simulink library "pathFollowingCtrlAoATurbFault_cl"  (R2020a)
settings: Solver=VariableStepAuto  StartTime=0.0  StopTime=10.0  RelTol=1e-3
undefined symbols (not defined in the file or in its folder): env, FLIGHTCONTROLLER, fltCtrl, initializeBussesFromBlock, lapN, pthCtrl1, rollVec, timeVec, tSwitch, VEHICLE, vhcl, yawVec
libraries: simulink x9, filteredPIDController_ul x4, vrlib x3, eulAng2RotMat_ul x2, alphaBeta_ul x2, velocityAngle_ul x2, filteredPIDControllerAWGS_ul x1, stopwatch_ul x1, tensionLimitCtrl_cl x1, courseFollowExp_cl x1, ctrlAllocMatrix3Comp_cl x1, angleBtw2Vecs_ul x1
settings Model: Creator=jldanie5  LastModifiedBy=andre
settings DataIOCC: ReturnWorkspaceOutputs=off
settings DebuggingCC: ArithmeticOperatorsInVariantConditions=warning
settings SFSimCC: CustomCodeUndefinedFunction=UseInterfaceOnly

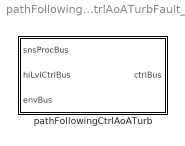
== system pathFollowingCtrlAoATurbFault_cl ==
  pathFollowingCtrlAoATurb : Subsystem  LoadFcn=initializeBussesFromBlock(gcb)  InitFcn=initializeBussesFromBlock(gcb)  StartFcn=initializeBussesFromBlock(gcb)  VariantControl=strcmpi(FLIGHTCONTROLLER,'pathFollowingControllerManta')  mask{initPosForInitSStar=vhcl.initPosVecGnd.Value, fluidDensity=env.water.density.Value, pathCtrl=pthCtrl1, aeroStruct=vhcl.struct('OCT.aeroSurf')}
      mask prompts: initPosForInitSStar "Initial Position"; fluidDensity "Fluid Density"; pathCtrl "Controller"; aeroStruct "Aerodynamic Structure"
      settings: MinAlgLoopOccurrences=on
      mask DialogControl Container3 Prompt: courseFollow Params
      mask DialogControl Container4 Prompt: setpointToOutput Params

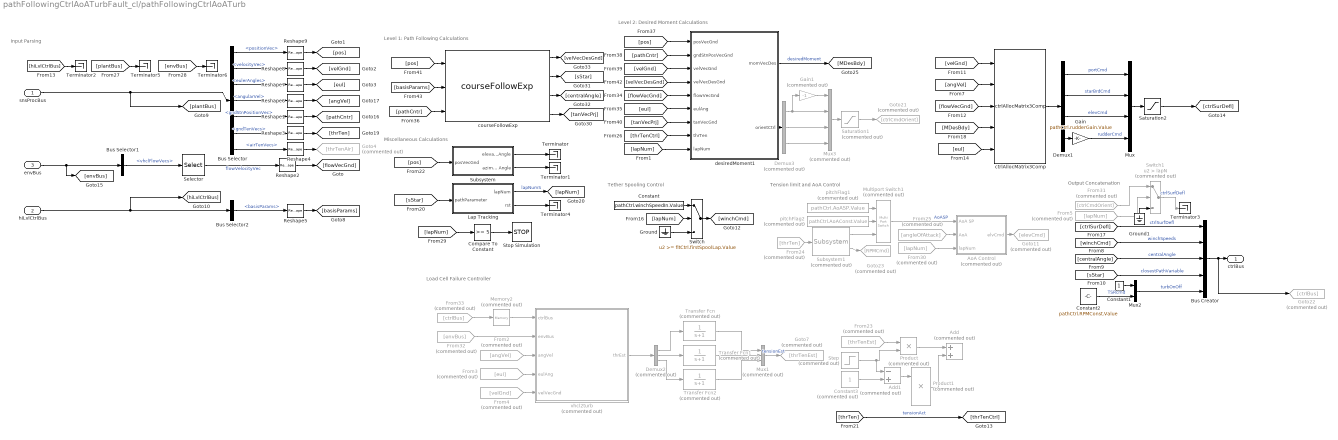
== system pathFollowingCtrlAoATurbFault_cl/pathFollowingCtrlAoATurb ==
  note: Load Cell Failure Controller
  note: Tension limit and AoA Control
  note: Miscellaneous Calculations
  note: Output Concatenation
  note: Tether Spooling Control
  note: Input Parsing
  note: Level 1: Path Following Calculations
  note: Level 2: Desired Moment Calculations
  snsProcBus : Inport  OutDataTypeStr=Bus: sensorsProcessingBus
  hiLvlCtrlBus : Inport  Port=2  OutDataTypeStr=Bus: hiLvlCtrlBus
  envBus : Inport  Port=3  OutDataTypeStr=Bus: envBus
  Add : Sum  Commented=on
  Add1 : Sum  Commented=on  Inputs=-+
  AoA Control : Subsystem  Commented=on
  Bus Creator : BusCreator  Inputs=5
  Bus Selector : BusSelector  OutputSignals=positionVec,velocityVec,eulerAngles,angularVel,gndStnPositionVec,gndTenVecs,airTenVecs
  Bus Selector1 : BusSelector  OutputSignals=vhclFlowVecs
  Bus Selector2 : BusSelector  OutputSignals=basisParams
  Compare To Constant : simulink/Logic and Bit Operations/Compare To Constant  relop=>=  const=5  OutDataTypeStr=boolean
  Constant : Constant  Value=pathCtrl.winchSpeedIn.Value
  Constant1 : Constant
  Constant2 : Constant  Value=pathCtrl.RPMConst.Value
  Constant3 : Constant  Commented=on
  Demux1 : Demux
  Demux2 : Demux  Commented=on  Outputs=3
  Demux3 : Demux  Commented=on  Outputs=3
  From2 : From  Commented=on  GotoTag=angVel
  From23 : From  Commented=on  GotoTag=thrTenEst
  From24 : From  Commented=on  GotoTag=thrTen
  From25 : From  Commented=on  GotoTag=angleOfAttack
  From3 : From  Commented=on  GotoTag=eul
  From30 : From  Commented=on  GotoTag=lapNum
  From31 : From  Commented=on  GotoTag=ctrlCmdOrient
  From32 : From  Commented=on  GotoTag=envBus
  From33 : From  Commented=on  GotoTag=ctrlBus
  From4 : From  Commented=on  GotoTag=velGnd
  From5 : From  Commented=on  GotoTag=lapNum
  Gain : Gain  Gain=pathCtrl.rudderGain.Value
  Gain1 : Gain  Commented=on  Gain=-1
  Goto11 : Goto  Commented=on  GotoTag=elevCmd
  Goto21 : Goto  Commented=on  GotoTag=ctrlCmdOrient
  Goto22 : Goto  Commented=on  GotoTag=ctrlBus
  Goto23 : Goto  Commented=on  GotoTag=RPMCmd
  Goto4 : Goto  Commented=on  GotoTag=thrTenAir
  Goto7 : Goto  Commented=on  GotoTag=thrTenEst
  Ground : Ground
  Ground1 : Ground
  Lap Tracking : Subsystem
  Memory2 : Memory  Commented=on  InitialCondition=pathCtrl.initPathVar.Value
  Multiport Switch1 : MultiPortSwitch  Commented=on  DataPortOrder=Specify indices  Inputs=2  DataPortIndices={0,1}
  Mux : Mux
  Mux1 : Mux  Commented=on  Inputs=3
  Mux2 : Mux  Inputs=2
  Mux3 : Mux  Commented=on
  Product : Product  Commented=on
  Product1 : Product  Commented=on
  Reshape{1..9} (9 alike) : Reshape  OutputDimensionality=Column vector (2-D)
  Saturation1 : Saturate  Commented=on  UpperLimit=pathCtrl.controlSigMax.upperLimit.Value  LowerLimit=pathCtrl.controlSigMax.lowerLimit.Value
  Saturation2 : Saturate  UpperLimit=pathCtrl.controlSigMax.upperLimit.Value  LowerLimit=pathCtrl.controlSigMax.lowerLimit.Value
  Selector : Selector  NumberOfDimensions=2  InputPortWidth=3  IndexOptions=Select all,Index vector (dialog)  Indices=[1 3],5  OutputSizes=1,1
  Step : Step  Commented=on  Time=tSwitch  SampleTime=0
  Stop Simulation : Stop
  Subsystem : Subsystem
  Subsystem1 : tensionLimitCtrl_cl/Subsystem  Commented=on  SystemSampleTime=-1  Latency=0  AutoFrameSizeCalculation=off
  Switch : Switch  Threshold=fltCtrl.firstSpoolLap.Value
  Switch1 : Switch  Commented=on  Criteria=u2 > Threshold  Threshold=lapN
  Terminator{,1..6} (7 alike) : Terminator
  Transfer Fcn : TransferFcn  Commented=on  Denominator=[1 1]
  Transfer Fcn1 : TransferFcn  Commented=on  Denominator=[1 1]
  Transfer Fcn2 : TransferFcn  Commented=on  Denominator=[1 1]
  courseFollowExp : courseFollowExp_cl/courseFollowExp  SystemSampleTime=-1  Latency=0  AutoFrameSizeCalculation=off
  ctrlAllocMatrix3Comp : ctrlAllocMatrix3Comp_cl/ctrlAllocMatrix3Comp  aeroStruct=vhcl.struct('OCT.aeroSurf')  fluidDensity=fluidDensity  arms=vhcl.struct('OCT.thrAttch')
  desiredMoment1 : Subsystem
  pitchFlag1 : Constant  Commented=on  Value=pathCtrl.AoASP.Value
  pitchFlag2 : Constant  Commented=on  Value=pathCtrl.AoAConst.Value
  vhcl2turb : Subsystem  Commented=on  VariantControl=strcmpi(VEHICLE,'vhcl2turb')  mask{vcl=vhcl, rho=env.water.density.Value, grav=env.gravAccel.Value}
      mask prompts: vcl "Vehicle"; rho "Density"; grav "Gravity"
      mask DialogControl Container9 Prompt: General
      mask DialogControl Container5 Prompt: Vehicle object (OCT.vehicle)
      mask DialogControl ParameterGroupVar Prompt: Environment Object (OCT.env)
      mask Display:
      | image('kite2.PNG',[0 0 700 700]/4,'on')
      | 
      | port_label('input',1,'ctrlBus')
      | port_label('input',2,'envBus')
      | port_label('input',3,'nodeForceVecs')
      | 
      | port_label('output',1,'thrTension')
  ctrlBus : Outport  OutDataTypeStr=Bus: fltCtrlBus  VectorParamsAs1DForOutWhenUnconnected=off
  wires:
  Bus Selector/6 -> Reshape3/1  "<gndTenVecs>"
  Reshape3/1 -> [thrTen]
  snsProcBus/1 -> Bus Selector/1, [plantBus]
  Bus Selector/2 -> Reshape8/1  "<velocityVec>"
  Bus Selector/1 -> Reshape9/1  "<positionVec>"
  Bus Selector/3 -> Reshape7/1  "<eulerAngles>"
  Bus Creator/1 -> Goto22/1, ctrlBus/1
  [winchCmd] -> Bus Creator/2  "winchSpeeds"
  hiLvlCtrlBus/1 -> [hiLvlCtrlBus], Bus Selector2/1
  [centralAngle] -> Bus Creator/3  "centralAngle"
  [sStar] -> Bus Creator/4  "closestPathVariable"
  Bus Selector/4 -> Reshape6/1  "<angularVel>"
  [angVel] -> ctrlAllocMatrix3Comp/2
  [velGnd] -> ctrlAllocMatrix3Comp/1
  [flowVecGnd] -> ctrlAllocMatrix3Comp/3
  Demux1/1 -> Mux/1  "portCmd"
  Demux1/2 -> Mux/2  "starBrdCmd"
  [MDesBdy] -> ctrlAllocMatrix3Comp/4
  [ctrlSurDefl] -> Bus Creator/1  "ctrlSurfDefl"
  Bus Selector2/1 -> Reshape5/1  "<basisParams>"
  Reshape5/1 -> [basisParams]
  Saturation2/1 -> [ctrlSurDefl]
  Reshape2/1 -> [flowVecGnd]
  Reshape6/1 -> [angVel]
  Reshape7/1 -> [eul]
  Reshape8/1 -> [velGnd]
  Reshape9/1 -> [pos]
  [eul] -> ctrlAllocMatrix3Comp/5
  Selector/1 -> Reshape2/1  "flowVelocityVec"
  envBus/1 -> [envBus], Bus Selector1/1
  Bus Selector1/1 -> Selector/1  "<vhclFlowVecs>"
  Reshape1/1 -> [pathCntr]
  Bus Selector/5 -> Reshape1/1  "<gndStnPositionVec>"
  Demux1/4 -> Gain/1
  [pos] -> Subsystem/1(posVecGnd)
  Subsystem/1(elevationAngle) -> Terminator/1
  Subsystem/2(azimuth Angle) -> Terminator1/1
  [sStar] -> Lap Tracking/1(pathParameter)
  Lap Tracking/2(rst) -> Terminator4/1
  Lap Tracking/1(lapNum) -> [lapNum]  "lapNumS"
  [plantBus] -> Terminator5/1
  [envBus] -> Terminator6/1
  Switch/1 -> [winchCmd]
  [lapNum] -> Switch/2
  Constant/1 -> Switch/1
  Ground/1 -> Switch/3
  [lapNum] -> Compare To Constant/1
  Compare To Constant/1 -> Stop Simulation/1
  ctrlAllocMatrix3Comp/1 -> Demux1/1
  Gain/1 -> Mux/4  "rudderCmd"
  [hiLvlCtrlBus] -> Terminator2/1
  From30/1 -> AoA Control/3(lapNum)
  AoA Control/1(elvCmd) -> Goto11/1
  From25/1 -> AoA Control/2(AoA)
  Mux/1 -> Saturation2/1
  Subsystem1/1 -> Multiport Switch1/3
  pitchFlag2/1 -> Multiport Switch1/2
  pitchFlag1/1 -> Multiport Switch1/1
  From24/1 -> Subsystem1/1
  Multiport Switch1/1 -> AoA Control/1(AoA SP)  "AoASP"
  Subsystem1/2 -> Goto23/1
  Mux2/1 -> Bus Creator/5  "turbOnOff"
  Constant1/1 -> Mux2/1
  Constant2/1 -> Mux2/2  "TSRcmd"
  Demux1/3 -> Mux/3  "elevCmd"
  [velVecDesGnd] -> desiredMoment1/4(velVecDesGnd)
  [velGnd] -> desiredMoment1/3(velVecGnd)
  [eul] -> desiredMoment1/6(eulAng)
  [basisParams] -> courseFollowExp/2
  [pathCntr] -> desiredMoment1/2(gndStnPosVecGnd)
  courseFollowExp/2 -> [sStar]
  [pos] -> desiredMoment1/1(posVecGnd)
  [tanVecPrj] -> desiredMoment1/7(tanVecGnd)
  [pathCntr] -> courseFollowExp/3
  desiredMoment1/1(momVecDes) -> [MDesBdy]  "desiredMoment"
  [pos] -> courseFollowExp/1
  courseFollowExp/3 -> [centralAngle]
  courseFollowExp/4 -> [tanVecPrj]
  courseFollowExp/1 -> [velVecDesGnd]
  [flowVecGnd] -> desiredMoment1/5(flowVecGnd)
  [thrTenCtrl] -> desiredMoment1/8(thrTen)
  Reshape4/1 -> Goto4/1
  Bus Selector/7 -> Reshape4/1  "<airTenVecs>"
  From23/1 -> Product/1
  [thrTen] -> [thrTenCtrl]  "tensionAct"
  Step/1 -> Product/2, Add1/1
  Product/1 -> Add/1
  Constant3/1 -> Add1/2
  Add1/1 -> Product1/1
  Product1/1 -> Add/2
  Mux1/1 -> Goto7/1  "tensionEst"
  Demux2/1 -> Transfer Fcn/1
  Demux2/2 -> Transfer Fcn1/1
  Demux2/3 -> Transfer Fcn2/1
  Transfer Fcn/1 -> Mux1/1
  Transfer Fcn1/1 -> Mux1/2
  Transfer Fcn2/1 -> Mux1/3
  desiredMoment1/2(orientCtrl) -> Demux3/1
  Demux3/1 -> Gain1/1, Mux3/2
  Gain1/1 -> Mux3/1
  Demux3/2 -> Mux3/3
  Mux3/1 -> Saturation1/1
  From31/1 -> Switch1/1
  From5/1 -> Switch1/2
  Switch1/1 -> Terminator3/1  "ctrlSurfDefl"
  Saturation1/1 -> Goto21/1
  From32/1 -> vhcl2turb/2(envBus)
  From33/1 -> Memory2/1
  Memory2/1 -> vhcl2turb/1(ctrlBus)
  vhcl2turb/1(thrEst) -> Demux2/1
  From2/1 -> vhcl2turb/3(angVel)
  From3/1 -> vhcl2turb/4(eulAng)
  From4/1 -> vhcl2turb/5(velVecGnd)
  Demux3/3 -> Mux3/4
  [lapNum] -> desiredMoment1/9(lapNum)
  Ground1/1 -> Switch1/3

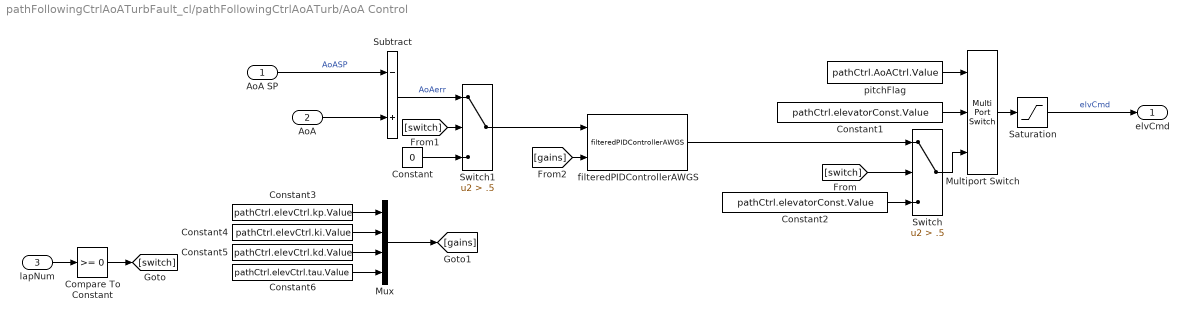
== system pathFollowingCtrlAoATurbFault_cl/pathFollowingCtrlAoATurb/AoA Control ==
  AoA SP : Inport
  AoA : Inport  Port=2
  lapNum : Inport  Port=3
  Compare To Constant : simulink/Logic and Bit Operations/Compare To Constant  relop=>=  const=0  OutDataTypeStr=boolean
  Constant : Constant  Value=0
  Constant1 : Constant  Value=pathCtrl.elevatorConst.Value
  Constant2 : Constant  Value=pathCtrl.elevatorConst.Value
  Constant3 : Constant  Value=pathCtrl.elevCtrl.kp.Value
  Constant4 : Constant  Value=pathCtrl.elevCtrl.ki.Value
  Constant5 : Constant  Value=pathCtrl.elevCtrl.kd.Value
  Constant6 : Constant  Value=pathCtrl.elevCtrl.tau.Value
  Multiport Switch : MultiPortSwitch  DataPortOrder=Specify indices  Inputs=2  DataPortIndices={0,1}
  Mux : Mux
  Saturation : Saturate  UpperLimit=pathCtrl.elevCtrlMax.upperLimit.Value  LowerLimit=pathCtrl.elevCtrlMax.lowerLimit.Value
  Subtract : Sum  Inputs=-+
  Switch : Switch  Criteria=u2 > Threshold  Threshold=.5
  Switch1 : Switch  Criteria=u2 > Threshold  Threshold=.5
  filteredPIDControllerAWGS : filteredPIDControllerAWGS_ul/filteredPIDControllerAWGS  cmax=pathCtrl.elevCtrlMax.upperLimit.Value  cmin=pathCtrl.elevCtrlMax.lowerLimit.Value
  pitchFlag : Constant  Value=pathCtrl.AoACtrl.Value
  elvCmd : Outport
  wires:
  AoA/1 -> Subtract/2
  Constant1/1 -> Multiport Switch/2
  pitchFlag/1 -> Multiport Switch/1
  AoA SP/1 -> Subtract/1  "AoASP"
  Multiport Switch/1 -> Saturation/1
  Constant2/1 -> Switch/3
  Saturation/1 -> elvCmd/1  "elvCmd"
  lapNum/1 -> Compare To Constant/1
  Compare To Constant/1 -> [switch]
  [switch] -> Switch/2
  Subtract/1 -> Switch1/1  "AoAerr"
  [switch] -> Switch1/2
  Constant/1 -> Switch1/3
  Switch/1 -> Multiport Switch/3
  Switch1/1 -> filteredPIDControllerAWGS/1
  filteredPIDControllerAWGS/1 -> Switch/1
  [gains] -> filteredPIDControllerAWGS/2
  Mux/1 -> [gains]
  Constant3/1 -> Mux/1
  Constant4/1 -> Mux/2
  Constant5/1 -> Mux/3
  Constant6/1 -> Mux/4

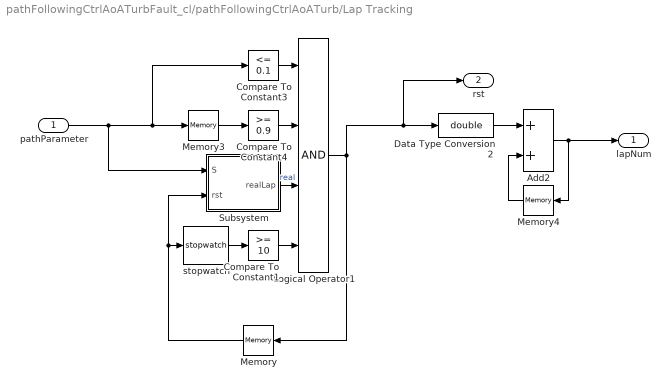
== system pathFollowingCtrlAoATurbFault_cl/pathFollowingCtrlAoATurb/Lap Tracking ==
  pathParameter : Inport
  Add2 : Sum
  Compare To Constant1 : simulink/Logic and Bit Operations/Compare To Constant  relop=>=  const=10  OutDataTypeStr=boolean
  Compare To Constant3 : simulink/Logic and Bit Operations/Compare To Constant  relop=<=  const=0.1  OutDataTypeStr=boolean
  Compare To Constant4 : simulink/Logic and Bit Operations/Compare To Constant  relop=>=  const=0.9  OutDataTypeStr=boolean
  Data Type Conversion2 : DataTypeConversion  OutDataTypeStr=double
  Logical Operator1 : Logic  Inputs=4  AllPortsSameDT=off  OutDataTypeStr=boolean
  Memory : Memory  InitialCondition=false
  Memory3 : Memory
  Memory4 : Memory
  Subsystem : Subsystem
  stopwatch : stopwatch_ul/stopwatch  SystemSampleTime=-1  Latency=0  AutoFrameSizeCalculation=off
  lapNum : Outport  VectorParamsAs1DForOutWhenUnconnected=off
  rst : Outport  Port=2  VectorParamsAs1DForOutWhenUnconnected=off
  wires:
  Compare To Constant3/1 -> Logical Operator1/1
  Memory3/1 -> Compare To Constant4/1
  Data Type Conversion2/1 -> Add2/1
  Logical Operator1/1 -> rst/1, Data Type Conversion2/1, Memory/1
  Memory4/1 -> Add2/2
  Add2/1 -> lapNum/1, Memory4/1
  Compare To Constant4/1 -> Logical Operator1/2
  pathParameter/1 -> Subsystem/1(S), Compare To Constant3/1, Memory3/1
  stopwatch/1 -> Compare To Constant1/1
  Memory/1 -> Subsystem/2(rst), stopwatch/1
  Compare To Constant1/1 -> Logical Operator1/4
  Subsystem/1(realLap) -> Logical Operator1/3  "real"

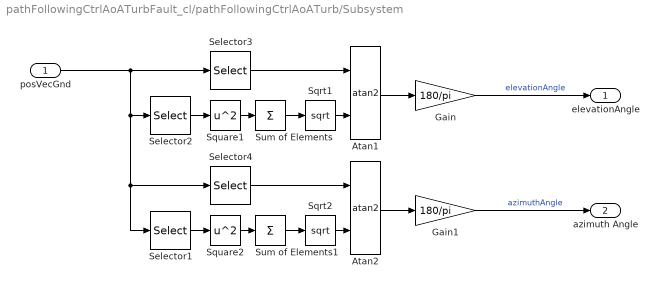
== system pathFollowingCtrlAoATurbFault_cl/pathFollowingCtrlAoATurb/Subsystem ==
  posVecGnd : Inport
  Atan1 : Trigonometry  Operator=atan2
  Atan2 : Trigonometry  Operator=atan2
  Gain : Gain  Gain=180/pi
  Gain1 : Gain  Gain=180/pi
  Selector1 : Selector  InputPortWidth=3  IndexOptions=Index vector (dialog)  Indices=1  OutputSizes=1
  Selector2 : Selector  InputPortWidth=3  IndexOptions=Index vector (dialog)  Indices=[1 2]  OutputSizes=1
  Selector3 : Selector  InputPortWidth=3  IndexOptions=Index vector (dialog)  Indices=3  OutputSizes=1
  Selector4 : Selector  InputPortWidth=3  IndexOptions=Index vector (dialog)  Indices=2  OutputSizes=1
  Sqrt1 : Sqrt  SaturateOnIntegerOverflow=on
  Sqrt2 : Sqrt  SaturateOnIntegerOverflow=on
  Square1 : Math  Operator=square  SignedPower=on  SaturateOnIntegerOverflow=on
  Square2 : Math  Operator=square  SignedPower=on  SaturateOnIntegerOverflow=on
  Sum of Elements : Sum  Inputs=+
  Sum of Elements1 : Sum  Inputs=+
  elevationAngle : Outport
  azimuth Angle : Outport  Port=2
  wires:
  Sqrt1/1 -> Atan1/2
  Square1/1 -> Sum of Elements/1
  Selector3/1 -> Atan1/1
  Sum of Elements/1 -> Sqrt1/1
  Atan1/1 -> Gain/1
  Selector2/1 -> Square1/1
  Gain/1 -> elevationAngle/1  "elevationAngle"
  Atan2/1 -> Gain1/1
  Square2/1 -> Sum of Elements1/1
  Sum of Elements1/1 -> Sqrt2/1
  Selector1/1 -> Square2/1
  posVecGnd/1 -> Selector1/1, Selector4/1, Selector2/1, Selector3/1
  Sqrt2/1 -> Atan2/2
  Selector4/1 -> Atan2/1
  Gain1/1 -> azimuth Angle/1  "azimuthAngle"

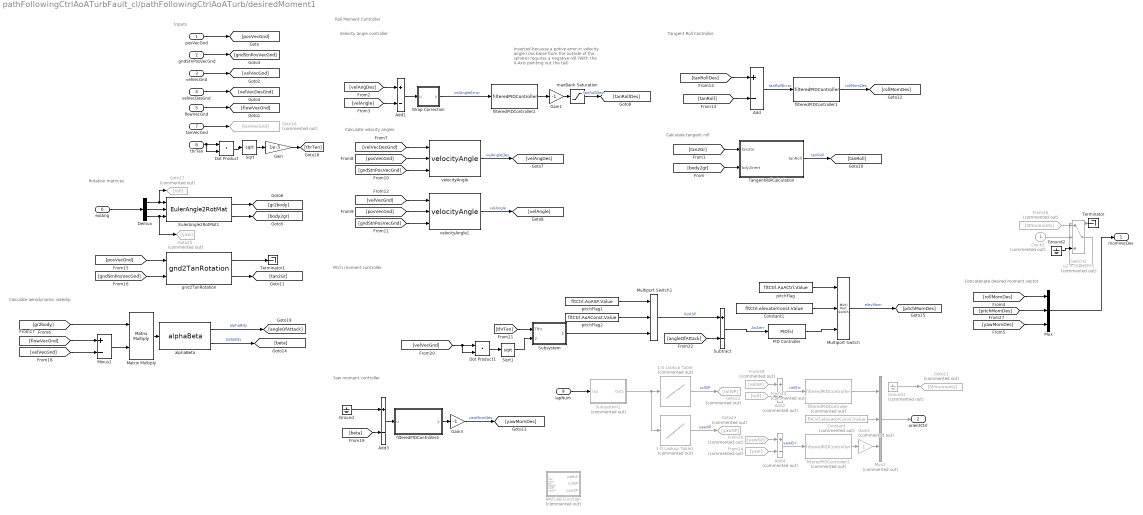
== system pathFollowingCtrlAoATurbFault_cl/pathFollowingCtrlAoATurb/desiredMoment1 ==
  note: Roll Moment Controller
  note: Calculate aerodynamic sideslip
  note: Concatenate desired moment vector
  note: Tangent Roll Controller
  note: Calculate tangent roll
  note: Calculate velocity angles
  note: Rotation matrices
  note: Inputs
  note: Velocity angle controller
  note: Inverted because a potive error
      | in velocity angle (clockwise from the
      | outside of the sphere) requires a negative
      | roll (With the X-Axis pointing out the tail)
  note: Pitch moment controller
  note: Yaw moment controller
  posVecGnd : Inport
  gndStnPosVecGnd : Inport  Port=2
  velVecGnd : Inport  Port=3
  velVecDesGnd : Inport  Port=4
  flowVecGnd : Inport  Port=5
  eulAng : Inport  Port=6
  tanVecGnd : Inport  Port=7
  thrTen : Inport  Port=8
  lapNum : Inport  Port=9
  1-D Lookup Table : Lookup_n-D  Commented=on  NumberOfTableDimensions=1  BreakpointsForDimension1=timeVec  Table=rollVec  InternalRulePriority=Speed  RndMeth=Simplest  InputSameDT=on
  1-D Lookup Table1 : Lookup_n-D  Commented=on  NumberOfTableDimensions=1  BreakpointsForDimension1=timeVec  Table=yawVec  InternalRulePriority=Speed  RndMeth=Simplest  InputSameDT=on
  Add : Sum  Inputs=+-
  Add1 : Sum  Inputs=+-
  Add2 : Sum  Commented=on  Inputs=+-
  Add3 : Sum  Inputs=+-
  Add4 : Sum  Commented=on  Inputs=+-
  Clock2 : Clock  Commented=on
  Constant : Constant  Commented=on  Value=fltCtrl.elevatorConst.Value
  Constant1 : Constant  Value=fltCtrl.elevatorConst.Value
  Demux : Demux  Outputs=3
  Dot Product : DotProduct  InputSameDT=on  OutDataTypeStr=Inherit: Inherit via internal rule
  Dot Product1 : DotProduct  InputSameDT=on  OutDataTypeStr=Inherit: Inherit via internal rule
  EulerAngle2RotMat1 : eulAng2RotMat_ul/EulerAngle2RotMat  SystemSampleTime=-1  Latency=0  AutoFrameSizeCalculation=off
  From23 : From  Commented=on  GotoTag=roll
  From24 : From  Commented=on  GotoTag=yaw
  From26 : From  Commented=on  GotoTag=SPmoments
  From28 : From  Commented=on  GotoTag=rollSP
  From29 : From  Commented=on  GotoTag=yawSP
  Gain : Gain  Gain=1e-3
  Gain1 : Gain  Gain=-1
  Gain3 : Gain  Gain=-1
  Gain5 : Gain  Commented=on  Gain=-1
  Goto16 : Goto  Commented=on  GotoTag=tanVecGnd
  Goto17 : Goto  Commented=on  GotoTag=roll
  Goto20 : Goto  Commented=on  GotoTag=yaw
  Goto21 : Goto  Commented=on  GotoTag=SPmoments
  Goto22 : Goto  Commented=on  GotoTag=rollSP
  Goto23 : Goto  Commented=on  GotoTag=yawSP
  Ground : Ground
  Ground1 : Ground  Commented=on
  Ground2 : Ground
  MATLAB Function : MATLAB Function  Commented=on  TreatAsAtomicUnit=on
  Matrix Multiply : Product  Multiplication=Matrix(*)
  Minus1 : Sum  Inputs=+-
  Multiport Switch : MultiPortSwitch  DataPortOrder=Specify indices  Inputs=2  DataPortIndices={0,1}
  Multiport Switch1 : MultiPortSwitch  DataPortOrder=Specify indices  Inputs=2  DataPortIndices={0,1}
  Mux : Mux  Inputs=3
  Mux2 : Mux  Commented=on  Inputs=3
  PID Controller : simulink/Continuous/PID Controller  Controller=PID  Form=Parallel  TimeDomain=Continuous-time  UseExternalTs=off  SampleTime=-1  IntegratorMethod=Forward Euler  FilterMethod=Forward Euler  ControllerParametersSource=internal  P=fltCtrl.pitchMoment.kp.Value  I=fltCtrl.pitchMoment.ki.Value  D=fltCtrl.pitchMoment.kd.Value  UseFilter=on  N=fltCtrl.pitchMoment.tau.Value  TunerSelectOption=Transfer Function Based (PID Tuner App)  InitialConditionSource=internal  InitialConditionForIntegrator=0  InitialConditionForFilter=0  DifferentiatorICPrevScaledInput=0  ExternalReset=none  TrackingMode=off  Kt=1  LimitOutput=off  UpperSaturationLimit=inf  LowerSaturationLimit=-100  LinearizeAsGain=on  AntiWindupMode=clamping  Kb=1  POutMin=[]  POutMax=[]  IOutMin=[]  IOutMax=[]  DOutMin=[]  DOutMax=[]  NOutMin=[]  NOutMax=[]  SumOutMin=[]  SumOutMax=[]  SaturationOutMin=[]  SaturationOutMax=[]  PParamMin=[]  PParamMax=[]  IParamMin=[]  IParamMax=[]  DParamMin=[]  DParamMax=[]  NParamMin=[]  NParamMax=[]  KbParamMin=[]  KbParamMax=[]  KtParamMin=[]  KtParamMax=[]  KbOutMin=[]  KbOutMax=[]  KtOutMin=[]  KtOutMax=[]  IntegratorOutMin=[]  IntegratorOutMax=[]  FilterOutMin=[]  FilterOutMax=[]  SumI1OutMin=[]  SumI1OutMax=[]  SumI2OutMin=[]  SumI2OutMax=[]  SumI3OutMin=[]  SumI3OutMax=[]  SumI4OutMin=[]  SumI4OutMax=[]  SumDOutMin=[]  SumDOutMax=[]  DifferentiatorOutMin=[]  DifferentiatorOutMax=[]  FilterDiffOutCoefMin=[]  FilterDiffOutCoefMax=[]  ReciprocalOutMin=[]  ReciprocalOutMax=[]  SumDenOutMin=[]  SumDenOutMax=[]  SumNumOutMin=[]  SumNumOutMax=[]  DivideOutMin=[]  DivideOutMax=[]  UdiffTsProdOutMin=[]  UdiffTsProdOutMax=[]  NTsProdOutMin=[]  NTsProdOutMax=[]  UintegralTsProdOutMin=[]  UintegralTsProdOutMax=[]  UngainTsProdOutMin=[]  UngainTsProdOutMax=[]  IntegratorContinuousStateAttributes=''  IntegratorStateMustResolveToSignalObject=off  IntegratorRTWStateStorageClass=Auto  FilterContinuousStateAttributes=''  FilterStateMustResolveToSignalObject=off  FilterRTWStateStorageClass=Auto  ParallelPVariant=InternalParameters  IdealPVariant=Disabled  IVariant=InternalParameters  DVariant=InternalParameters  IntegratorVariant=Continuous  SatVariant=Disabled  AWVariant=Passthrough  PCopyVariant=Disabled  TRVariant=Disabled  FdbkBlocksVariant=Forward  IdealPFdbkVariant=Disabled  SatFdbkVariant=Disabled  DerivativeFilterVariant=ContFilter  NVariant=InternalParameters  NCopyVariant=Disabled  FilterICVariant=InternalICsFilter  IntegratorICVariant=InternalICs  ExternalResetVariant=Disabled  TRSumVariant=Passthrough  SumFdbkVariant=Disabled  SumVariant=Sum_PID  TsampFilterVariant=InternalTs  TsampNgainVariant=Passthrough  TsampIntegralVariant=Passthrough
  Sqrt : Sqrt  SaturateOnIntegerOverflow=on
  Sqrt1 : Sqrt  SaturateOnIntegerOverflow=on
  Subsystem : Subsystem
  Subsystem1 : Subsystem  Commented=on
  Subtract : Sum  Inputs=+-
  Switch2 : Switch  Commented=on  Criteria=u2 > Threshold  Threshold=tSwitch*5
  TangentRollCalculation : Subsystem
  Terminator : Terminator
  Terminator1 : Terminator
  Wrap Correction : Subsystem
  alphaBeta : alphaBeta_ul/alphaBeta  SystemSampleTime=-1  Latency=0  AutoFrameSizeCalculation=off
  filteredPIDController : filteredPIDController_ul/filteredPIDController  Commented=on  kp=fltCtrl.rollCtrl.kp.Value  ki=fltCtrl.rollCtrl.ki.Value  kd=fltCtrl.rollCtrl.kd.Value  Value=fltCtrl.rollCtrl.tau.Value  externalReset=none
  filteredPIDController1 : filteredPIDController_ul/filteredPIDController  kp=pathCtrl.rollMoment.kp.Value  ki=0  kd=pathCtrl.rollMoment.kd.Value  Value=pathCtrl.rollMoment.tau.Value  externalReset=none
  filteredPIDController2 : filteredPIDController_ul/filteredPIDController  kp=pathCtrl.tanRoll.kp.Value  ki=pathCtrl.tanRoll.ki.Value  kd=pathCtrl.tanRoll.kd.Value  Value=pathCtrl.tanRoll.tau.Value  externalReset=none
  filteredPIDController3 : filteredPIDController_ul/filteredPIDController  Commented=on  kp=fltCtrl.yawCtrl.kp.Value  ki=fltCtrl.yawCtrl.ki.Value  kd=fltCtrl.yawCtrl.kd.Value  Value=fltCtrl.yawCtrl.tau.Value  externalReset=none
  filteredPIDController4 : Subsystem  mask{kp=pathCtrl.yawMoment.kp.Value, ki=0, kd=pathCtrl.yawMoment.kd.Value, Value=pathCtrl.yawMoment.tau.Value, externalReset=none}
      mask prompts: kp "Proportional Gain, kp"; ki "Integral Gain, ki"; kd "Derivative Gain, kd"; Value "Time Constant, s"; externalReset "External reset:"
      mask init:
      | initfcn
      mask TypeOptions kp: kp/Gain
      mask TypeOptions ki: ki/Gain
      mask TypeOptions kd: kd/Gain
      mask TypeOptions Value: tau/Value
      mask TypeOptions externalReset: none | rising | falling | either | level | level hold
  gnd2TanRotation : gnd2TanRotation_ul/gnd2TanRotation  SystemSampleTime=-1  Latency=0  AutoFrameSizeCalculation=off
  maxBank Saturation : Saturate  UpperLimit=pathCtrl.maxBank.upperLimit.Value  LowerLimit=pathCtrl.maxBank.lowerLimit.Value
  pitchFlag : Constant  Value=fltCtrl.AoACtrl.Value
  pitchFlag1 : Constant  Value=fltCtrl.AoASP.Value
  pitchFlag2 : Constant  Value=fltCtrl.AoAConst.Value
  velocityAngle : velocityAngle_ul/velocityAngle  SystemSampleTime=-1  Latency=0  AutoFrameSizeCalculation=off
  velocityAngle1 : velocityAngle_ul/velocityAngle  SystemSampleTime=-1  Latency=0  AutoFrameSizeCalculation=off
  momVecDes : Outport  VectorParamsAs1DForOutWhenUnconnected=off
  orientCtrl : Outport  Port=2
  wires:
  filteredPIDController1/1 -> [rollMomDes]  "rollMomDes"
  [rollMomDes] -> Mux/1
  Wrap Correction/1(y) -> filteredPIDController2/1  "velAngleError"
  tanVecGnd/1 -> Goto16/1
  posVecGnd/1 -> [posVecGnd]
  velVecGnd/1 -> [velVecGnd]
  Add/1 -> filteredPIDController1/1  "tanRollError"
  Gain1/1 -> maxBank Saturation/1
  maxBank Saturation/1 -> [tanRollDes]  "tanRollDes"
  Add1/1 -> Wrap Correction/1(u)
  flowVecGnd/1 -> [flowVecGnd]
  [tan2Gr] -> TangentRollCalculation/1(tan2Gr)
  TangentRollCalculation/1(tanRoll) -> [tanRoll]  "tanRoll"
  Minus1/1 -> Matrix Multiply/2
  [velVecGnd] -> Minus1/2
  [flowVecGnd] -> Minus1/1
  eulAng/1 -> Demux/1
  Demux/2 -> EulerAngle2RotMat1/2
  EulerAngle2RotMat1/2 -> [body2gr]
  EulerAngle2RotMat1/1 -> [gr2body]
  [body2gr] -> TangentRollCalculation/2(bdy2Inert)
  [gr2body] -> Matrix Multiply/1
  Matrix Multiply/1 -> alphaBeta/1
  alphaBeta/2 -> [beta]  "betaBdy"
  alphaBeta/1 -> [angleOfAttack]  "alphaBdy"
  gndStnPosVecGnd/1 -> [gndStnPosVecGnd]
  velVecDesGnd/1 -> [velVecDesGnd]
  velocityAngle/1 -> [velAngDes]  "velAngleDes"
  velocityAngle1/1 -> [velAngle]  "velAngle"
  [velAngDes] -> Add1/1
  [velAngle] -> Add1/2
  [velVecDesGnd] -> velocityAngle/1
  [posVecGnd] -> velocityAngle/2
  [posVecGnd] -> velocityAngle1/2
  [gndStnPosVecGnd] -> velocityAngle/3
  [gndStnPosVecGnd] -> velocityAngle1/3
  [velVecGnd] -> velocityAngle1/1
  [tanRoll] -> Add/2
  [tanRollDes] -> Add/1
  [posVecGnd] -> gnd2TanRotation/1
  [gndStnPosVecGnd] -> gnd2TanRotation/2
  gnd2TanRotation/2 -> [tan2Gr]
  gnd2TanRotation/1 -> Terminator1/1
  [yawMomDes] -> Mux/3
  filteredPIDController2/1 -> Gain1/1
  [beta] -> Add3/2
  Ground/1 -> Add3/1
  Add3/1 -> filteredPIDController4/1(u)
  filteredPIDController4/1(y) -> Gain3/1
  Subsystem/1(AoA SP) -> Multiport Switch1/3
  [thrTen] -> Subsystem/1(Tthr)
  pitchFlag1/1 -> Multiport Switch1/1
  pitchFlag2/1 -> Multiport Switch1/2
  [pitchMomDes] -> Mux/2
  Gain3/1 -> [yawMomDes]  "yawMomDes"
  Multiport Switch/1 -> [pitchMomDes]  "elevMom"
  pitchFlag/1 -> Multiport Switch/1
  [angleOfAttack] -> Subtract/2
  Constant1/1 -> Multiport Switch/2
  PID Controller/1 -> Multiport Switch/3
  Subtract/1 -> PID Controller/1  "AoAerr"
  thrTen/1 -> Dot Product/2, Dot Product/1
  Sqrt/1 -> Gain/1
  Dot Product/1 -> Sqrt/1
  Gain/1 -> [thrTen]
  [velVecGnd] -> Dot Product1/2, Dot Product1/1
  Sqrt1/1 -> Subsystem/2(vAppSqr)
  Dot Product1/1 -> Sqrt1/1
  From24/1 -> Add4/2
  Mux2/1 -> orientCtrl/1
  filteredPIDController3/1 -> Gain5/1
  Gain5/1 -> Mux2/3
  Add4/1 -> filteredPIDController3/1  "yawErr"
  From23/1 -> Add2/2
  Add2/1 -> filteredPIDController/1  "rollErr"
  filteredPIDController/1 -> Mux2/1
  Demux/1 -> Goto17/1, EulerAngle2RotMat1/1
  Demux/3 -> Goto20/1, EulerAngle2RotMat1/3
  From26/1 -> Switch2/1
  Switch2/1 -> Terminator/1
  Clock2/1 -> Switch2/2
  Mux/1 -> momVecDes/1
  Multiport Switch1/1 -> Subtract/1  "AoASP"
  Constant/1 -> Mux2/2
  Ground1/1 -> Goto21/1
  From28/1 -> Add2/1
  From29/1 -> Add4/1
  1-D Lookup Table/1 -> Goto22/1  "rollSP"
  1-D Lookup Table1/1 -> Goto23/1  "yawSP"
  Subsystem1/1(Out1) -> 1-D Lookup Table1/1, 1-D Lookup Table/1
  lapNum/1 -> Subsystem1/1(lap)
  Ground2/1 -> Switch2/3

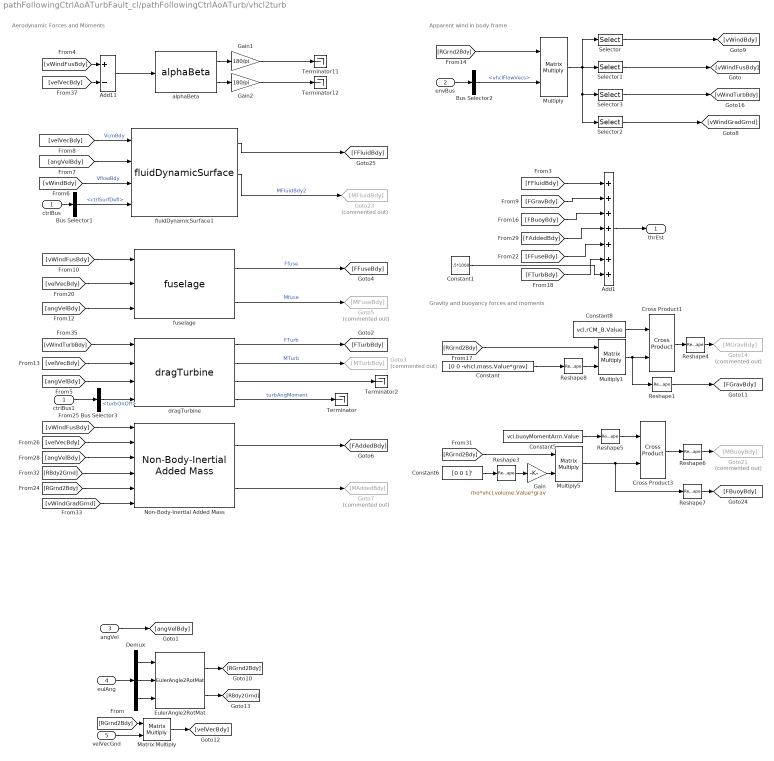
== system pathFollowingCtrlAoATurbFault_cl/pathFollowingCtrlAoATurb/vhcl2turb ==
  note: Aerodynamic Forces and Moments
  note: Gravity and buoyancy forces and moments
  note: Apparent wind in body frame
  ctrlBus : Inport  OutDataTypeStr=Bus: fltCtrlBus
  envBus : Inport  Port=2  OutDataTypeStr=Bus: envBus
  angVel : Inport  Port=3
  eulAng : Inport  Port=4
  velVecGnd : Inport  Port=5
  Add1 : Sum  Inputs=+++++++
  Add11 : Sum  Inputs=+-
  Bus Selector1 : BusSelector  OutputSignals=ctrlSurfDefl
  Bus Selector2 : BusSelector  OutputSignals=vhclFlowVecs
  Bus Selector3 : BusSelector  OutputSignals=turbOnOff
  Constant : Constant  Value=[0 0 -vhcl.mass.Value*grav]
  Constant1 : Constant  Value=.5*1000
  Constant5 : Constant  Value=vcl.buoyMomentArm.Value
  Constant6 : Constant  Value=[0 0 1]'
  Constant8 : Constant  Value=vcl.rCM_B.Value
  Cross Product1 : vrlib/Utilities/Cross Product
  Cross Product3 : vrlib/Utilities/Cross Product
  Demux : Demux  Outputs=3
  EulerAngle2RotMat : eulAng2RotMat_ul/EulerAngle2RotMat  SystemSampleTime=-1  Latency=0  AutoFrameSizeCalculation=off
  Gain : Gain  Gain=rho*vhcl.volume.Value*grav
  Gain1 : Gain  Gain=180/pi
  Gain2 : Gain  Gain=180/pi
  Goto14 : Goto  Commented=on  GotoTag=MGravBdy
  Goto21 : Goto  Commented=on  GotoTag=MBuoyBdy
  Goto23 : Goto  Commented=on  GotoTag=MFluidBdy
  Goto3 : Goto  Commented=on  GotoTag=MTurbBdy
  Goto5 : Goto  Commented=on  GotoTag=MFuseBdy
  Goto7 : Goto  Commented=on  GotoTag=MAddedBdy
  Matrix Multiply : Product  Multiplication=Matrix(*)
  Multiply : Product  Multiplication=Matrix(*)
  Multiply1 : Product  Multiplication=Matrix(*)
  Multiply5 : Product  Multiplication=Matrix(*)
  Non-Body-Inertial Added Mass : addedMass_cl/Non-Body-Inertial Added Mass  MaMat=vcl.Ma6x6_LE.Value  rB_LE=vcl.rB_LE.Value  gradDist=vcl.flowGradientDist.Value
  Reshape{1,3..8} (7 alike) : Reshape  OutputDimensionality=Column vector (2-D)
  Selector : Selector  NumberOfDimensions=2  InputPortWidth=3  IndexOptions=Select all,Index vector (dialog)  Indices=[1 3],1:4  OutputSizes=1,1
  Selector1 : Selector  NumberOfDimensions=2  InputPortWidth=3  IndexOptions=Select all,Index vector (dialog)  Indices=[1 3],5  OutputSizes=1,1
  Selector2 : Selector  NumberOfDimensions=2  InputPortWidth=3  IndexOptions=Select all,Index vector (dialog)  Indices=[1 3],8:13  OutputSizes=1,1
  Selector3 : Selector  NumberOfDimensions=2  InputPortWidth=3  IndexOptions=Select all,Index vector (dialog)  Indices=[1 3],6:7  OutputSizes=1,1
  Terminator{,2,11..12} (4 alike) : Terminator
  alphaBeta : alphaBeta_ul/alphaBeta  SystemSampleTime=-1  Latency=0  AutoFrameSizeCalculation=off
  ctrlBus1 : InportShadow  OutDataTypeStr=Bus: fltCtrlBus
  dragTurbine : dragTurbineNew_ul/dragTurbine  SystemSampleTime=-1  Latency=0  AutoFrameSizeCalculation=off
  fluidDynamicSurface1 : Copy_of_fluidDynamicSurface_cl/fluidDynamicSurface  vcl=vcl  fluidDensity=env.water.density.Value  fluidMomentArms=vcl.fluidMomentArms.Value  fluidRefArea=vcl.fluidRefArea.Value  wingTips=vcl.wingTipPositions.Value
  fuselage : fuselage_cl/fuselage  momArm=vcl.fuseMomentArm.Value  fus=vcl.fuse  fusRhoDa=rho
  thrEst : Outport
  wires:
  dragTurbine/4 -> Terminator/1  "turbAngMoment"
  [velVecBdy] -> fluidDynamicSurface1/1  "VcmBdy"
  [angVelBdy] -> fluidDynamicSurface1/2
  [vWindBdy] -> fluidDynamicSurface1/3  "VflowBdy"
  Bus Selector1/1 -> fluidDynamicSurface1/4  "<ctrlSurfDefl>"
  fluidDynamicSurface1/2 -> Goto23/1  "MFluidBdy2"
  fluidDynamicSurface1/1 -> [FFluidBdy]
  Gain2/1 -> Terminator12/1
  alphaBeta/1 -> Gain1/1
  Gain1/1 -> Terminator11/1
  alphaBeta/2 -> Gain2/1
  [velVecBdy] -> Add11/2
  Add11/1 -> alphaBeta/1
  [vWindFusBdy] -> Add11/1
  Non-Body-Inertial Added Mass/2 -> Goto7/1
  Non-Body-Inertial Added Mass/1 -> [FAddedBdy]
  Selector3/1 -> [vWindTurbBdy]
  ctrlBus1/1 -> Bus Selector3/1
  Bus Selector3/1 -> dragTurbine/4  "<turbOnOff>"
  Add1/1 -> thrEst/1
  [FAddedBdy] -> Add1/4
  [FTurbBdy] -> Add1/6
  [FFuseBdy] -> Add1/5
  [FBuoyBdy] -> Add1/3
  [FGravBdy] -> Add1/2
  [FFluidBdy] -> Add1/1
  Selector2/1 -> [vWindGradGrnd]
  Selector1/1 -> [vWindFusBdy]
  Selector/1 -> [vWindBdy]
  Multiply/1 -> Selector1/1, Selector3/1, Selector2/1, Selector/1
  Bus Selector2/1 -> Multiply/2  "<vhclFlowVecs>"
  envBus/1 -> Bus Selector2/1
  [RGrnd2Bdy] -> Multiply/1
  Reshape4/1 -> Goto14/1
  Cross Product1/1 -> Reshape4/1
  Constant8/1 -> Cross Product1/1
  Reshape8/1 -> Multiply1/2
  [RGrnd2Bdy] -> Multiply1/1
  Constant/1 -> Reshape8/1
  fuselage/2 -> Goto5/1  "Mfuse"
  fuselage/1 -> [FFuseBdy]  "Ffuse"
  Multiply1/1 -> Cross Product1/2, Reshape1/1
  Reshape1/1 -> [FGravBdy]
  Reshape7/1 -> [FBuoyBdy]
  Multiply5/1 -> Cross Product3/2, Reshape7/1
  Reshape6/1 -> Goto21/1
  Cross Product3/1 -> Reshape6/1
  Reshape5/1 -> Cross Product3/1
  Constant5/1 -> Reshape5/1
  Gain/1 -> Multiply5/2
  [RGrnd2Bdy] -> Multiply5/1
  Reshape3/1 -> Gain/1
  Constant6/1 -> Reshape3/1
  [vWindGradGrnd] -> Non-Body-Inertial Added Mass/6
  [RGrnd2Bdy] -> Non-Body-Inertial Added Mass/5
  [RBdy2Grnd] -> Non-Body-Inertial Added Mass/4
  [angVelBdy] -> Non-Body-Inertial Added Mass/3
  [velVecBdy] -> Non-Body-Inertial Added Mass/2
  [vWindFusBdy] -> Non-Body-Inertial Added Mass/1
  dragTurbine/3 -> Terminator2/1
  dragTurbine/2 -> Goto3/1  "MTurb"
  dragTurbine/1 -> [FTurbBdy]  "FTurb"
  [angVelBdy] -> dragTurbine/3
  [velVecBdy] -> dragTurbine/2
  [vWindTurbBdy] -> dragTurbine/1
  [angVelBdy] -> fuselage/3
  [velVecBdy] -> fuselage/2
  [vWindFusBdy] -> fuselage/1
  ctrlBus/1 -> Bus Selector1/1
  Demux/3 -> EulerAngle2RotMat/3
  eulAng/1 -> Demux/1
  EulerAngle2RotMat/1 -> [RGrnd2Bdy]
  Demux/1 -> EulerAngle2RotMat/1
  Demux/2 -> EulerAngle2RotMat/2
  angVel/1 -> [angVelBdy]
  [RGrnd2Bdy] -> Matrix Multiply/1
  velVecGnd/1 -> Matrix Multiply/2
  Matrix Multiply/1 -> [velVecBdy]
  EulerAngle2RotMat/2 -> [RBdy2Grnd]
  Constant1/1 -> Add1/7

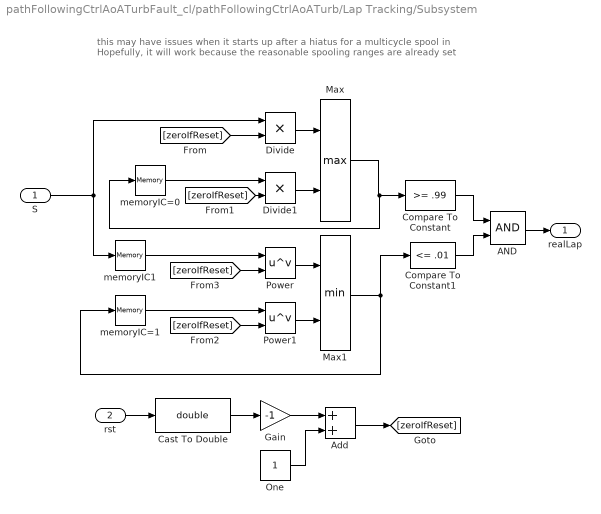
== system pathFollowingCtrlAoATurbFault_cl/pathFollowingCtrlAoATurb/Lap Tracking/Subsystem ==
  note: this may have issues when it starts up after a hiatus for a multicycle spool in
      | Hopefully, it will work because the reasonable spooling ranges are already set
  S : Inport
  rst : Inport  Port=2
  AND : Logic  AllPortsSameDT=off  OutDataTypeStr=boolean
  Add : Sum
  Cast To Double : DataTypeConversion  OutDataTypeStr=double
  Compare To Constant : simulink/Logic and Bit Operations/Compare To Constant  relop=>=  const=.99  OutDataTypeStr=boolean
  Compare To Constant1 : simulink/Logic and Bit Operations/Compare To Constant  relop=<=  const=.01  OutDataTypeStr=boolean
  Divide : Product  Inputs=**
  Divide1 : Product  Inputs=**
  Gain : Gain  Gain=-1
  Max : MinMax  Function=max  Inputs=2
  Max1 : MinMax  Inputs=2
  One : Constant  OutDataTypeStr=Inherit: Inherit via back propagation
  Power : Math  Operator=pow  SaturateOnIntegerOverflow=on
  Power1 : Math  Operator=pow  SaturateOnIntegerOverflow=on
  memoryIC1 : Memory  InitialCondition=1
  memoryIC=0 : Memory
  memoryIC=1 : Memory  InitialCondition=1
  realLap : Outport
  wires:
  Max1/1 -> Compare To Constant1/1, memoryIC=1/1
  rst/1 -> Cast To Double/1
  S/1 -> Divide/1, memoryIC1/1
  Gain/1 -> Add/1
  Add/1 -> [zeroIfReset]
  One/1 -> Add/2
  Divide/1 -> Max/1
  Max/1 -> memoryIC=0/1, Compare To Constant/1
  Power/1 -> Max1/1
  Power1/1 -> Max1/2
  Cast To Double/1 -> Gain/1
  Compare To Constant/1 -> AND/1
  Compare To Constant1/1 -> AND/2
  AND/1 -> realLap/1
  [zeroIfReset] -> Divide/2
  [zeroIfReset] -> Power/2
  [zeroIfReset] -> Divide1/2
  Divide1/1 -> Max/2
  memoryIC=0/1 -> Divide1/1
  [zeroIfReset] -> Power1/2
  memoryIC=1/1 -> Power1/1
  memoryIC1/1 -> Power/1

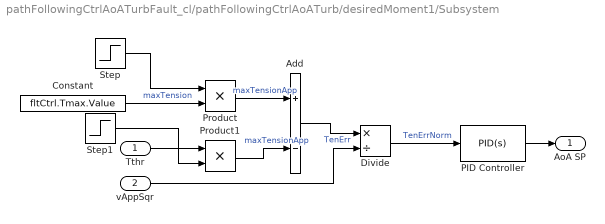
== system pathFollowingCtrlAoATurbFault_cl/pathFollowingCtrlAoATurb/desiredMoment1/Subsystem ==
  Tthr : Inport
  vAppSqr : Inport  Port=2
  Add : Sum  Inputs=+-
  Constant : Constant  Value=fltCtrl.Tmax.Value
  Divide : Product  Inputs=*/
  PID Controller : simulink/Continuous/PID Controller  Controller=PID  Form=Parallel  TimeDomain=Continuous-time  UseExternalTs=off  SampleTime=-1  IntegratorMethod=Forward Euler  FilterMethod=Forward Euler  ControllerParametersSource=internal  P=fltCtrl.alphaCtrl.kp.Value  I=fltCtrl.alphaCtrl.ki.Value  D=fltCtrl.alphaCtrl.kd.Value  UseFilter=on  N=fltCtrl.alphaCtrl.tau.Value  TunerSelectOption=Transfer Function Based (PID Tuner App)  InitialConditionSource=internal  InitialConditionForIntegrator=0  InitialConditionForFilter=0  DifferentiatorICPrevScaledInput=0  ExternalReset=none  TrackingMode=off  Kt=1  LimitOutput=on  UpperSaturationLimit=fltCtrl.AoAConst.Value  LowerSaturationLimit=fltCtrl.AoAmin.Value  LinearizeAsGain=on  AntiWindupMode=clamping  Kb=1  POutMin=[]  POutMax=[]  IOutMin=[]  IOutMax=[]  DOutMin=[]  DOutMax=[]  NOutMin=[]  NOutMax=[]  SumOutMin=[]  SumOutMax=[]  SaturationOutMin=[]  SaturationOutMax=[]  PParamMin=[]  PParamMax=[]  IParamMin=[]  IParamMax=[]  DParamMin=[]  DParamMax=[]  NParamMin=[]  NParamMax=[]  KbParamMin=[]  KbParamMax=[]  KtParamMin=[]  KtParamMax=[]  KbOutMin=[]  KbOutMax=[]  KtOutMin=[]  KtOutMax=[]  IntegratorOutMin=[]  IntegratorOutMax=[]  FilterOutMin=[]  FilterOutMax=[]  SumI1OutMin=[]  SumI1OutMax=[]  SumI2OutMin=[]  SumI2OutMax=[]  SumI3OutMin=[]  SumI3OutMax=[]  SumI4OutMin=[]  SumI4OutMax=[]  SumDOutMin=[]  SumDOutMax=[]  DifferentiatorOutMin=[]  DifferentiatorOutMax=[]  FilterDiffOutCoefMin=[]  FilterDiffOutCoefMax=[]  ReciprocalOutMin=[]  ReciprocalOutMax=[]  SumDenOutMin=[]  SumDenOutMax=[]  SumNumOutMin=[]  SumNumOutMax=[]  DivideOutMin=[]  DivideOutMax=[]  UdiffTsProdOutMin=[]  UdiffTsProdOutMax=[]  NTsProdOutMin=[]  NTsProdOutMax=[]  UintegralTsProdOutMin=[]  UintegralTsProdOutMax=[]  UngainTsProdOutMin=[]  UngainTsProdOutMax=[]  IntegratorContinuousStateAttributes=''  IntegratorStateMustResolveToSignalObject=off  IntegratorRTWStateStorageClass=Auto  FilterContinuousStateAttributes=''  FilterStateMustResolveToSignalObject=off  FilterRTWStateStorageClass=Auto  ParallelPVariant=InternalParameters  IdealPVariant=Disabled  IVariant=InternalParameters  DVariant=InternalParameters  IntegratorVariant=Continuous  SatVariant=Enabled  AWVariant=ContClampingParallel  PCopyVariant=Disabled  TRVariant=Disabled  FdbkBlocksVariant=Forward  IdealPFdbkVariant=Disabled  SatFdbkVariant=Disabled  DerivativeFilterVariant=ContFilter  NVariant=InternalParameters  NCopyVariant=Disabled  FilterICVariant=InternalICsFilter  IntegratorICVariant=InternalICs  ExternalResetVariant=Disabled  TRSumVariant=Passthrough  SumFdbkVariant=Disabled  SumVariant=Sum_PID  TsampFilterVariant=InternalTs  TsampNgainVariant=Passthrough  TsampIntegralVariant=Passthrough
  Product : Product
  Product1 : Product
  Step : Step  Time=tSwitch  Before=1  After=.9  SampleTime=0
  Step1 : Step  Time=0  Before=1  After=1.05  SampleTime=0
  AoA SP : Outport
  wires:
  Divide/1 -> PID Controller/1  "TenErrNorm"
  Constant/1 -> Product/2  "maxTension"
  PID Controller/1 -> AoA SP/1
  Add/1 -> Divide/1  "TenErr"
  vAppSqr/1 -> Divide/2
  Step/1 -> Product/1
  Product/1 -> Add/1  "maxTensionApp"
  Tthr/1 -> Product1/1
  Product1/1 -> Add/2  "maxTensionApp"
  Step1/1 -> Product1/2

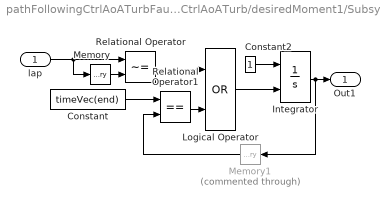
== system pathFollowingCtrlAoATurbFault_cl/pathFollowingCtrlAoATurb/desiredMoment1/Subsystem1 ==
  lap : Inport
  Constant : Constant  Value=timeVec(end)
  Constant2 : Constant
  Integrator : Integrator  ExternalReset=rising
  Logical Operator : Logic  Operator=OR  AllPortsSameDT=off  OutDataTypeStr=boolean
  Memory : Memory
  Memory1 : Memory  Commented=through
  Relational Operator : RelationalOperator  Operator=~=  OutDataTypeStr=boolean  RndMeth=Simplest
  Relational Operator1 : RelationalOperator  Operator===  OutDataTypeStr=boolean  RndMeth=Simplest
  Out1 : Outport
  wires:
  Memory/1 -> Relational Operator/2
  Constant2/1 -> Integrator/1
  lap/1 -> Memory/1, Relational Operator/1
  Integrator/1 -> Memory1/1, Out1/1
  Logical Operator/1 -> Integrator/2
  Relational Operator/1 -> Logical Operator/1
  Relational Operator1/1 -> Logical Operator/2
  Constant/1 -> Relational Operator1/1
  Memory1/1 -> Relational Operator1/2

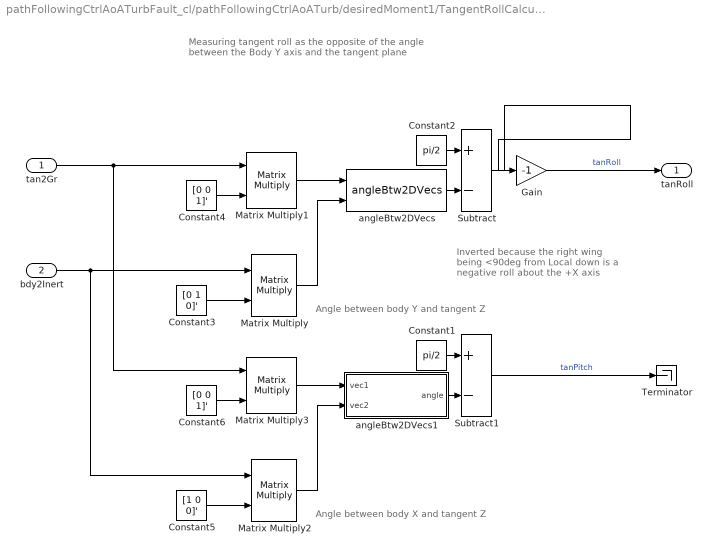
== system pathFollowingCtrlAoATurbFault_cl/pathFollowingCtrlAoATurb/desiredMoment1/TangentRollCalculation ==
  note: Measuring tangent roll as the opposite
      | of the angle between the Body Y axis
      | and the tangent plane
  note: Angle between body Y and tangent Z
  note: Inverted because the right wing
      | being <90deg from Local down
      | is a negative roll about the +X axis
  note: Angle between body X and tangent Z
  tan2Gr : Inport
  bdy2Inert : Inport  Port=2
  Constant1 : Constant  Value=pi/2
  Constant2 : Constant  Value=pi/2
  Constant3 : Constant  Value=[0 1 0]'
  Constant4 : Constant  Value=[0 0 1]'
  Constant5 : Constant  Value=[1 0 0]'
  Constant6 : Constant  Value=[0 0 1]'
  Gain : Gain  Gain=-1
  Matrix Multiply{,1..3} (4 alike) : Product  Multiplication=Matrix(*)
  Subtract : Sum  Inputs=+-
  Subtract1 : Sum  Inputs=+-
  Terminator : Terminator
  angleBtw2DVecs : angleBtw2Vecs_ul/angleBtw2DVecs  SystemSampleTime=-1  Latency=0  AutoFrameSizeCalculation=off
  angleBtw2DVecs1 : Subsystem
  tanRoll : Outport  VectorParamsAs1DForOutWhenUnconnected=off
  wires:
  Subtract/1 -> Gain/1
  Constant3/1 -> Matrix Multiply/2
  angleBtw2DVecs/1 -> Subtract/2
  Constant2/1 -> Subtract/1
  Matrix Multiply1/1 -> angleBtw2DVecs/1
  Constant4/1 -> Matrix Multiply1/2
  Matrix Multiply/1 -> angleBtw2DVecs/2
  Gain/1 -> tanRoll/1  "tanRoll"
  bdy2Inert/1 -> Matrix Multiply2/1, Matrix Multiply/1
  Subtract1/1 -> Terminator/1  "tanPitch"
  tan2Gr/1 -> Matrix Multiply3/1, Matrix Multiply1/1
  Matrix Multiply2/1 -> angleBtw2DVecs1/2(vec2)
  Constant6/1 -> Matrix Multiply3/2
  Matrix Multiply3/1 -> angleBtw2DVecs1/1(vec1)
  Constant1/1 -> Subtract1/1
  angleBtw2DVecs1/1(angle) -> Subtract1/2
  Constant5/1 -> Matrix Multiply2/2

== system pathFollowingCtrlAoATurbFault_cl/pathFollowingCtrlAoATurb/desiredMoment1/Wrap Correction ==
  note: output = mod(input-pi,2*pi)-pi
      | wraps output to -pi to pi
      |
      | ex) 1.5*pi will become -.5pi
      | 	and -1.5pi will become .5pi
      |
      | to visualize, plot the fuction above
  u : Inport
  Add1 : Sum  Inputs=+-
  Add2 : Sum  Inputs=+-
  Constant1 : Constant  Value=pi
  Constant2 : Constant  Value=2*pi
  Constant3 : Constant  Value=pi
  Mod : Math  Operator=mod  SignedPower=on  SaturateOnIntegerOverflow=on
  y : Outport  VectorParamsAs1DForOutWhenUnconnected=off
  wires:
  u/1 -> Add1/1
  Constant1/1 -> Add1/2
  Add1/1 -> Mod/1
  Constant2/1 -> Mod/2
  Mod/1 -> Add2/1  "always_pos"
  Constant3/1 -> Add2/2
  Add2/1 -> y/1

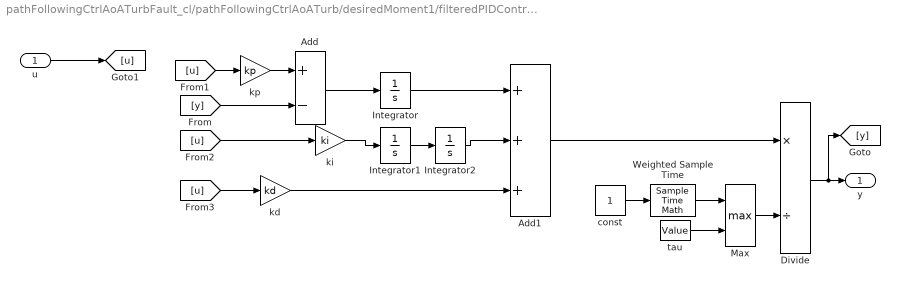
== system pathFollowingCtrlAoATurbFault_cl/pathFollowingCtrlAoATurb/desiredMoment1/filteredPIDController4 ==
  u : Inport  PortDimensions=1
  Add : Sum  Inputs=+-
  Add1 : Sum  Inputs=+++
  Divide : Product  Inputs=*/
  Integrator : Integrator
  Integrator1 : Integrator
  Integrator2 : Integrator
  Max : MinMax  Function=max  Inputs=2
  Weighted Sample Time : SampleTimeMath  TsampMathOp=Ts Only
  const : Constant
  kd : Gain  Gain=kd
  ki : Gain  Gain=ki
  kp : Gain  Gain=kp
  tau : Constant  Value=Value
  y : Outport  PortDimensions=1  VectorParamsAs1DForOutWhenUnconnected=off
  wires:
  u/1 -> [u]
  kp/1 -> Add/1
  [y] -> Add/2
  Add/1 -> Integrator/1
  [u] -> kp/1
  Max/1 -> Divide/2
  tau/1 -> Max/2
  Integrator1/1 -> Integrator2/1
  ki/1 -> Integrator1/1
  [u] -> ki/1
  [u] -> kd/1
  Integrator2/1 -> Add1/2
  Integrator/1 -> Add1/1
  kd/1 -> Add1/3
  Add1/1 -> Divide/1
  Divide/1 -> [y], y/1
  Weighted Sample Time/1 -> Max/1
  const/1 -> Weighted Sample Time/1

== system pathFollowingCtrlAoATurbFault_cl/pathFollowingCtrlAoATurb/desiredMoment1/TangentRollCalculation/angleBtw2DVecs1 ==
  vec1 : Inport
  vec2 : Inport  Port=2
  Abs : Abs
  Atan2 : Trigonometry  Operator=atan2
  Cross Product : vrlib/Utilities/Cross Product
      settings: SourceProductBaseCode=VR
  Dot Product : DotProduct  InputSameDT=on  OutDataTypeStr=Inherit: Inherit via internal rule
  Dot Product1 : DotProduct  InputSameDT=on  OutDataTypeStr=Inherit: Inherit via internal rule
  Sqrt : Sqrt  SaturateOnIntegerOverflow=on
  angle : Outport  VectorParamsAs1DForOutWhenUnconnected=off
  wires:
  Atan2/1 -> Abs/1
  vec1/1 -> Dot Product/1, Cross Product/2
  vec2/1 -> Cross Product/1, Dot Product/2
  Cross Product/1 -> Dot Product1/1, Dot Product1/2
  Dot Product/1 -> Atan2/2
  Abs/1 -> angle/1
  Dot Product1/1 -> Sqrt/1
  Sqrt/1 -> Atan2/1

== matlab function pathFollowingCtrlAoATurbFault_cl/pathFollowingCtrlAoATurb/desiredMoment1/MATLAB Function ==
  data: pathS output; s input; rollSP output; roll input; yaw input; en input; pathP input; rollP input; yawP input; yawSP output
function [pathS,rollSP,yawSP] = fcn(s,roll,yaw,en,pathP,rollP,yawP)

N = numel(pathP);
pathS = zeros(N,1);
rollSP = zeros(N,1);
yawSP = zeros(N,1);

if en == 1
    pathS = pathP;
    rollSP = rollP;
    yawSP = yawP;
else
    for i = 2:N
        pathS(i) = pathS(i-1);
    end
end
